simulink model "myLIN_F16Block"  (Simulink 7.6)
settings: Solver=ode5  StartTime=0.0  StopTime=100  FixedStep=0.001  RelTol=1e-3
values from neighbouring files (symbols this model uses):
  dLEF = 0    [F16Data.mat]    (also in F16LinmodTestData.m; F16NolinearModelInitialData.m; F16NolinearModelRemoveWindControlData_low.m; F16hi_7500_394_all.mat)
  fi_flag_Simulink = 0    [F16Data.mat]    (also in F16hi_7500_394_all.mat; F16lo_7500_394_all.mat; myFindF16Dynamics.m; runLINF16sim.m)
  trim_control_hi = [-2.97973164861 0.00874607850104 0.0680302158183]    [F16Data.mat]    (also in F16hi_7500_394_all.mat = [-1.41046812571 -0.0839337172095 -0.0125601395798]; F16lo_7500_394_all.mat = [-1.41046812571 -0.0839337172095 -0.0125601395798])
  trim_control_lo = [-1.5494258131 -1.24450697103e-10 -4.77959844983e-09]    [F16Data.mat]    (also in F16hi_7500_394_all.mat = [-1.08947517229 0.155794241881 0.128606760221]; F16lo_7500_394_all.mat = [-1.64183174326 -4.38546100082e-10 -1.68300124238e-08])
  trim_state_lin = [0 0 9843 0 1.13910469244e-17 0 393.72 1.13910469244e-17 0 0 0 0]    [F16Data.mat]    (also in F16hi_7500_394_all.mat = [0 0 7500 0 0.000279617532986 0 394 0.000279617532986 0 0 0 ; F16lo_7500_394_all.mat = [0 0 7500 0 0.0237311750075 0 394 0.0237311750075 0 0 0 0]; myFindF16Dynamics.m = trim_state_lo; runLINF16sim.m = trim_state_lo)
  trim_thrust_hi = 2279.08519955    [F16Data.mat]    (also in F16hi_7500_394_all.mat = -26942.451508; F16lo_7500_394_all.mat = -26942.451508)
  trim_thrust_lo = -206727.459732    [F16Data.mat]    (also in F16hi_7500_394_all.mat = 1004.07804585; F16lo_7500_394_all.mat = -98159.5668651)
settings Model: Creator=keviczky  LastModifiedBy=WhisPer  ExtModeAutoUpdateStatusClock=off
settings DataIOCC: Decimation=50  LimitDataPoints=off  SignalLoggingName=sigsOut
settings OptimizationCC: BooleanDataType=off
settings DebuggingCC: SaveWithParameterizedLinksMsg=none  SignalResolutionControl=TryResolveAllWithWarning  SolverPrmCheckMsg=none  MultiTaskDSMMsg=warning  MultiTaskCondExecSysMsg=none  StrictBusMsg=None
settings HardwareCC: TargetUnknown=on
settings RTWCC: IncludeERTFirstTime=on

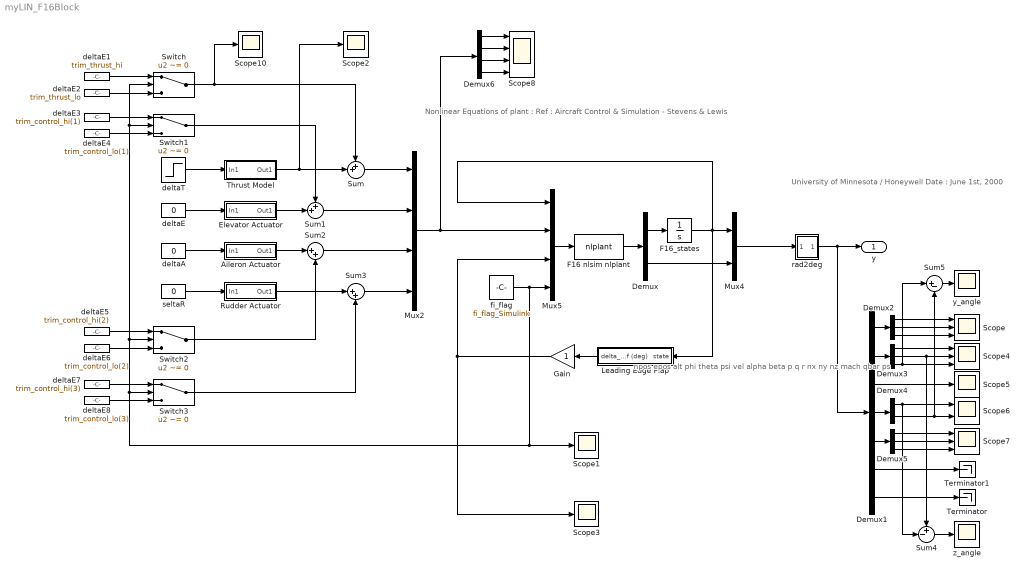
== system myLIN_F16Block ==
  note: npos
      | epos
      | alt
      | phi
      | theta
      | psi
      | vel
      | alpha
      | beta
      | p
      | q
      | r
      | nx
      | ny
      | nz
      | mach
      | qbar
      | ps
  note: University of Minnesota / Honeywell
      | Date : June 1st, 2000
  note: Nonlinear Equations of plant :
      | Ref : Aircraft Control & Simulation
      | - Stevens & Lewis
  Aileron Actuator : Subsystem  AncestorBlock=F16_Actuator_Library/Aileron Actuator
  Demux : Demux  Outputs=[12 6]
  Demux1 : Demux  Outputs=[3 3 1 2 3 3 3]
  Demux2 : Demux  Outputs=3
  Demux3 : Demux  Outputs=3
  Demux4 : Demux  Outputs=2
  Demux5 : Demux  Outputs=3
  Demux6 : Demux
  Elevator Actuator : Subsystem  AncestorBlock=F16_Actuator_Library/Elevator Actuator
  F16 nlsim nlplant : MATLABFcn  MATLABFcn=nlplant  OutputDimensions=18  OutputSignalType=real
  F16_states : Integrator  InitialCondition=trim_state_lin
  Gain : Gain
  Leading Edge Flap : Subsystem
  Mux2 : Mux
  Mux4 : Mux  Inputs=2
  Mux5 : Mux  Inputs=[12 4 1 1]
  Rudder Actuator : Subsystem  AncestorBlock=F16_Actuator_Library/Rudder Actuator
  Scope : Scope  NumInputPorts=3
      settings: YMin=-9000~-4e-008~2000  YMax=3000~1.6e-007~9500
  Scope{1..3,5,10} (5 alike) : Scope
      Scope1 settings: YMin=0  YMax=3500
      Scope10 settings: YMin=0  YMax=3500  SaveName=ScopeData12
      Scope2 settings: YMin=0  YMax=3500  SaveName=ScopeData2
      Scope3 settings: YMin=-13.5  YMax=-9  SaveName=ScopeData3
      Scope5 settings: YMin=-13.5  YMax=-9  SaveName=ScopeData5
  Scope4 : Scope  NumInputPorts=3
      settings: YMin=-9000~-4e-008~2000  YMax=3000~1.6e-007~9500  SaveName=ScopeData4
  Scope6 : Scope  NumInputPorts=2
      settings: YMin=-9000~-4e-008  YMax=3000~1.6e-007  SaveName=ScopeData6
  Scope7 : Scope  NumInputPorts=3
      settings: YMin=-9000~-4e-008~2000  YMax=3000~1.6e-007~9500  SaveName=ScopeData7
  Scope8 : Scope  NumInputPorts=4
      settings: YMin=-9000~-4e-008~2000~-5  YMax=3000~1.6e-007~9500~5  SaveName=ScopeData8
  Sum : Sum  Inputs=++|
  Sum1 : Sum  Inputs=++|
  Sum2 : Sum  Inputs=|++
  Sum3 : Sum  Inputs=|++
  Sum4 : Sum  Inputs=+-|
  Sum5 : Sum  Inputs=|+-
  Switch{,1..3} (4 alike) : Switch  Criteria=u2 ~= 0
  Terminator : Terminator
  Terminator1 : Terminator
  Thrust Model : Subsystem  AncestorBlock=F16_Actuator_Library/Thrust Model
  deltaA : Constant  Value=0
  deltaE : Constant  Value=0
  deltaE1 : Constant  Value=trim_thrust_hi
  deltaE2 : Constant  Value=trim_thrust_lo
  deltaE3 : Constant  Value=trim_control_hi(1)
  deltaE4 : Constant  Value=trim_control_lo(1)
  deltaE5 : Constant  Value=trim_control_hi(2)
  deltaE6 : Constant  Value=trim_control_lo(2)
  deltaE7 : Constant  Value=trim_control_hi(3)
  deltaE8 : Constant  Value=trim_control_lo(3)
  deltaT : Step  Time=5  After=0  SampleTime=0
  fi_flag : Constant  Value=fi_flag_Simulink
  rad2deg : Subsystem
  seltaR : Constant  Value=0
  y_angle : Scope
      settings: YMin=0  YMax=3500  SaveName=ScopeData10
  z_angle : Scope
      settings: YMin=0  YMax=3500  SaveName=ScopeData9
  y : Outport
  wires:
  Mux4/1 -> rad2deg/1(In1)
  F16 nlsim nlplant/1 -> Demux/1
  Demux/1 -> F16_states/1
  Demux/2 -> Mux4/2
  Mux5/1 -> F16 nlsim nlplant/1
  Mux2/1 -> Mux5/2, Demux6/1
  rad2deg/1(Out1) -> y/1, Demux1/1
  F16_states/1 -> Mux4/1, Mux5/1, Leading Edge Flap/1(state)
  fi_flag/1 -> Mux5/4, Scope1/1, Switch3/2, Switch2/2, Switch/2, Switch1/2
  Leading Edge Flap/1(delta_lef (deg)) -> Gain/1
  Demux1/1 -> Demux2/1
  Demux2/1 -> Scope/1
  Demux2/2 -> Scope/2
  Demux2/3 -> Scope/3
  Demux1/7 -> Terminator/1
  deltaE1/1 -> Switch/1
  deltaE2/1 -> Switch/3
  deltaE3/1 -> Switch1/1
  deltaE4/1 -> Switch1/3
  deltaE5/1 -> Switch2/1
  deltaE6/1 -> Switch2/3
  deltaE7/1 -> Switch3/1
  deltaE8/1 -> Switch3/3
  seltaR/1 -> Rudder Actuator/1(In1)
  deltaA/1 -> Aileron Actuator/1(In1)
  deltaE/1 -> Elevator Actuator/1(In1)
  deltaT/1 -> Thrust Model/1(In1)
  Elevator Actuator/1(Out1) -> Sum1/2
  Sum1/1 -> Mux2/2
  Sum/1 -> Mux2/1
  Thrust Model/1(Out1) -> Sum/2, Scope2/1
  Sum3/1 -> Mux2/4
  Rudder Actuator/1(Out1) -> Sum3/1
  Aileron Actuator/1(Out1) -> Sum2/1
  Sum2/1 -> Mux2/3
  Demux3/1 -> Scope4/1
  Demux3/2 -> Scope4/2, Sum4/1
  Demux3/3 -> Scope4/3, Sum5/1
  Demux1/2 -> Demux3/1
  Demux1/3 -> Scope5/1
  Demux1/4 -> Demux4/1
  Demux4/1 -> Scope6/1, Sum4/2
  Demux4/2 -> Scope6/2, Sum5/2
  Demux5/1 -> Scope7/1
  Demux5/2 -> Scope7/2
  Demux5/3 -> Scope7/3
  Demux1/5 -> Demux5/1
  Demux1/6 -> Terminator1/1
  Demux6/1 -> Scope8/1
  Demux6/2 -> Scope8/2
  Demux6/3 -> Scope8/3
  Demux6/4 -> Scope8/4
  Switch/1 -> Sum/1, Scope10/1
  Switch1/1 -> Sum1/1
  Sum4/1 -> z_angle/1
  Sum5/1 -> y_angle/1
  Gain/1 -> Mux5/3, Scope3/1
  Switch2/1 -> Sum2/2
  Switch3/1 -> Sum3/2

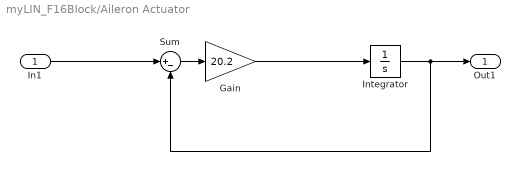
== system myLIN_F16Block/Aileron Actuator ==
  In1 : Inport
  Gain : Gain  Gain=20.2  SaturateOnIntegerOverflow=on  OutDataTypeStr=Inherit: Same as input  ParamDataTypeStr=Inherit: Same as input
  "Integrator " : Integrator  UpperSaturationLimit=21.5  LowerSaturationLimit=-21.5
  Sum : Sum  Inputs=|+-  SaturateOnIntegerOverflow=on  InputSameDT=on  OutDataTypeStr=Inherit: Same as first input
  Out1 : Outport
  wires:
  "Integrator "/1 -> Sum/2, Out1/1
  Gain/1 -> "Integrator "/1
  Sum/1 -> Gain/1
  In1/1 -> Sum/1

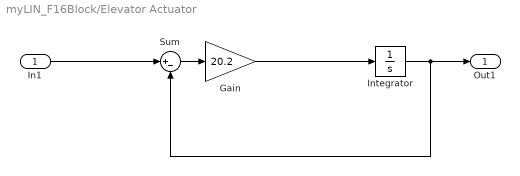
== system myLIN_F16Block/Elevator Actuator ==
  In1 : Inport
  Gain : Gain  Gain=20.2  SaturateOnIntegerOverflow=on  OutDataTypeStr=Inherit: Same as input  ParamDataTypeStr=Inherit: Same as input
  "Integrator " : Integrator  UpperSaturationLimit=25  LowerSaturationLimit=-25
  Sum : Sum  Inputs=|+-  SaturateOnIntegerOverflow=on  InputSameDT=on  OutDataTypeStr=Inherit: Same as first input
  Out1 : Outport
  wires:
  "Integrator "/1 -> Sum/2, Out1/1
  Gain/1 -> "Integrator "/1
  Sum/1 -> Gain/1
  In1/1 -> Sum/1

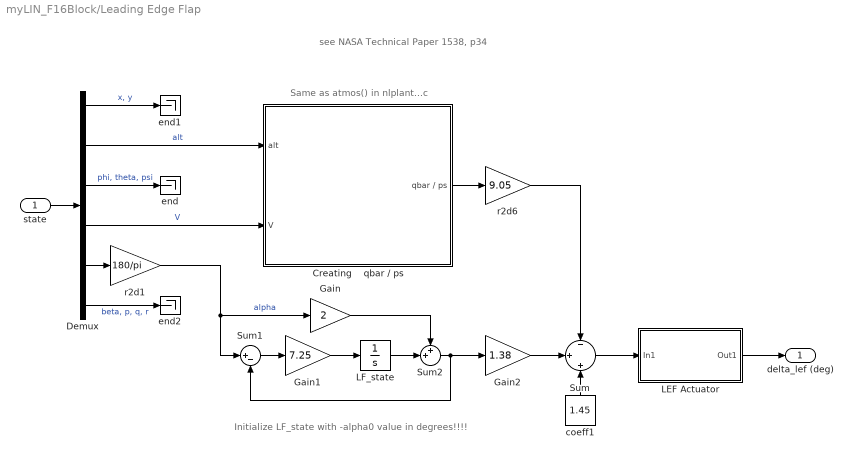
== system myLIN_F16Block/Leading Edge Flap ==
  note: see NASA Technical Paper 1538, p34
  note: Same as atmos() in nlplant...c
  note: Initialize LF_state with -alpha0 value in degrees!!!!
  state : Inport
  Creating    qbar / ps : Subsystem
  Demux : Demux  Outputs=[2,1,3,1,1,4]
  Gain : Gain  Gain=2  SaturateOnIntegerOverflow=on  OutDataTypeStr=Inherit: Same as input  ParamDataTypeStr=Inherit: Same as input
  Gain1 : Gain  Gain=7.25  SaturateOnIntegerOverflow=on  OutDataTypeStr=Inherit: Same as input  ParamDataTypeStr=Inherit: Same as input
  Gain2 : Gain  Gain=1.38  SaturateOnIntegerOverflow=on  OutDataTypeStr=Inherit: Same as input  ParamDataTypeStr=Inherit: Same as input
  LEF Actuator : Subsystem  AncestorBlock=F16_Actuator_Library/Aileron Actuator
  LF_state : Integrator  InitialCondition=-trim_state_lin(8)*180/pi
  Sum : Sum  Inputs=-|+|+  SaturateOnIntegerOverflow=on  InputSameDT=on  OutDataTypeStr=Inherit: Same as first input
  Sum1 : Sum  Inputs=|+-  SaturateOnIntegerOverflow=on  InputSameDT=on  OutDataTypeStr=Inherit: Same as first input
  Sum2 : Sum  Inputs=++|  SaturateOnIntegerOverflow=on  InputSameDT=on  OutDataTypeStr=Inherit: Same as first input
  coeff1 : Constant  Value=1.45
  end : Terminator
  end1 : Terminator
  end2 : Terminator
  r2d1 : Gain  Gain=180/pi  SaturateOnIntegerOverflow=on  OutDataTypeStr=Inherit: Same as input  ParamDataTypeStr=Inherit: Same as input
  r2d6 : Gain  Gain=9.05  SaturateOnIntegerOverflow=on  OutDataTypeStr=Inherit: Same as input  ParamDataTypeStr=Inherit: Same as input
  delta_lef (deg) : Outport
  wires:
  LEF Actuator/1(Out1) -> delta_lef (deg)/1
  Sum/1 -> LEF Actuator/1(In1)
  Demux/3 -> end/1  "phi, theta, psi"
  state/1 -> Demux/1
  Sum1/1 -> Gain1/1
  Gain1/1 -> LF_state/1
  Gain/1 -> Sum2/1
  Gain2/1 -> Sum/2
  Demux/1 -> end1/1  "x, y"
  Demux/5 -> r2d1/1
  Demux/6 -> end2/1  "beta, p, q, r"
  coeff1/1 -> Sum/3
  Sum2/1 -> Sum1/2, Gain2/1
  LF_state/1 -> Sum2/2
  r2d1/1 -> Sum1/1, Gain/1  "alpha"
  Demux/4 -> Creating    qbar / ps/2(V)  "V"
  Creating    qbar / ps/1(qbar / ps) -> r2d6/1
  r2d6/1 -> Sum/1
  Demux/2 -> Creating    qbar / ps/1(alt)  "alt"

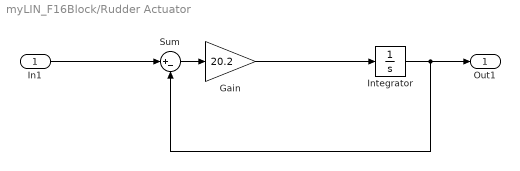
== system myLIN_F16Block/Rudder Actuator ==
  In1 : Inport
  Gain : Gain  Gain=20.2  SaturateOnIntegerOverflow=on  OutDataTypeStr=Inherit: Same as input  ParamDataTypeStr=Inherit: Same as input
  "Integrator " : Integrator  UpperSaturationLimit=30  LowerSaturationLimit=-30
  Sum : Sum  Inputs=|+-  SaturateOnIntegerOverflow=on  InputSameDT=on  OutDataTypeStr=Inherit: Same as first input
  Out1 : Outport
  wires:
  "Integrator "/1 -> Sum/2, Out1/1
  Gain/1 -> "Integrator "/1
  Sum/1 -> Gain/1
  In1/1 -> Sum/1

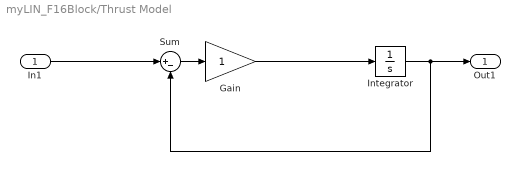
== system myLIN_F16Block/Thrust Model ==
  In1 : Inport
  Gain : Gain  SaturateOnIntegerOverflow=on  OutDataTypeStr=Inherit: Same as input  ParamDataTypeStr=Inherit: Same as input
  "Integrator " : Integrator  UpperSaturationLimit=30  LowerSaturationLimit=-30
  Sum : Sum  Inputs=|+-  SaturateOnIntegerOverflow=on  InputSameDT=on  OutDataTypeStr=Inherit: Same as first input
  Out1 : Outport
  wires:
  "Integrator "/1 -> Sum/2, Out1/1
  Gain/1 -> "Integrator "/1
  Sum/1 -> Gain/1
  In1/1 -> Sum/1

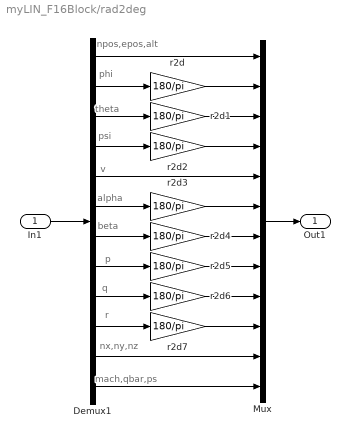
== system myLIN_F16Block/rad2deg ==
  note: npos,epos,alt
  note: phi
  note: theta
  note: psi
  note: v
  note: alpha
  note: beta
  note: p
  note: q
  note: r
  note: nx,ny,nz
  note: mach,qbar,ps
  In1 : Inport
  Demux1 : Demux  Outputs=[3 1 1 1 1 1 1 1 1 1 3 3]
  Mux : Mux  Inputs=[3 1 1 1 1 1 1 1 1 1 3 3]
  r2d{,1..7} (8 alike) : Gain  Gain=180/pi  SaturateOnIntegerOverflow=on  OutDataTypeStr=Inherit: Same as input  ParamDataTypeStr=Inherit: Same as input
  Out1 : Outport
  wires:
  In1/1 -> Demux1/1
  Demux1/2 -> r2d/1
  Demux1/3 -> r2d1/1
  Demux1/4 -> r2d2/1
  Demux1/1 -> Mux/1
  Demux1/5 -> Mux/5
  r2d2/1 -> Mux/4
  r2d1/1 -> Mux/3
  r2d/1 -> Mux/2
  Demux1/6 -> r2d3/1
  Demux1/7 -> r2d4/1
  Demux1/8 -> r2d5/1
  Demux1/9 -> r2d6/1
  Demux1/10 -> r2d7/1
  r2d3/1 -> Mux/6
  r2d4/1 -> Mux/7
  r2d5/1 -> Mux/8
  r2d6/1 -> Mux/9
  r2d7/1 -> Mux/10
  Mux/1 -> Out1/1
  Demux1/11 -> Mux/11
  Demux1/12 -> Mux/12

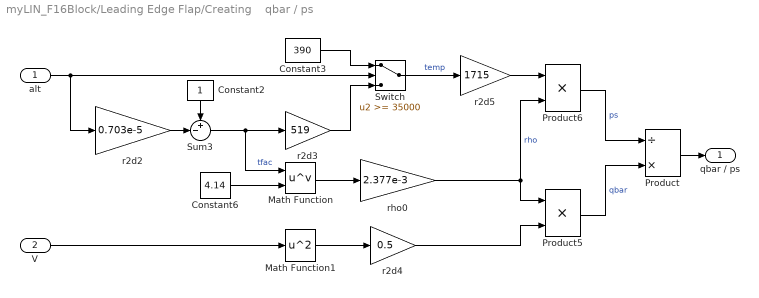
== system myLIN_F16Block/Leading Edge Flap/Creating    qbar / ps ==
  alt : Inport
  V : Inport  Port=2
  Constant2 : Constant
  Constant3 : Constant  Value=390
  Constant6 : Constant  Value=4.14
  Math Function : Math  Operator=pow  SaturateOnIntegerOverflow=on
  Math Function1 : Math  Operator=square  SaturateOnIntegerOverflow=on
  Product : Product  Inputs=/*  SaturateOnIntegerOverflow=on  InputSameDT=on  OutDataTypeStr=Inherit: Same as first input
  Product5 : Product  Inputs=**  SaturateOnIntegerOverflow=on  InputSameDT=on  OutDataTypeStr=Inherit: Same as first input
  Product6 : Product  Inputs=**  SaturateOnIntegerOverflow=on  InputSameDT=on  OutDataTypeStr=Inherit: Same as first input
  Sum3 : Sum  Inputs=+-|  SaturateOnIntegerOverflow=on  InputSameDT=on  OutDataTypeStr=Inherit: Same as first input
  Switch : Switch  Threshold=35000  SaturateOnIntegerOverflow=on  InputSameDT=on
  r2d2 : Gain  Gain=0.703e-5  SaturateOnIntegerOverflow=on  OutDataTypeStr=Inherit: Same as input  ParamDataTypeStr=Inherit: Same as input
  r2d3 : Gain  Gain=519  SaturateOnIntegerOverflow=on  OutDataTypeStr=Inherit: Same as input  ParamDataTypeStr=Inherit: Same as input
  r2d4 : Gain  Gain=0.5  SaturateOnIntegerOverflow=on  OutDataTypeStr=Inherit: Same as input  ParamDataTypeStr=Inherit: Same as input
  r2d5 : Gain  Gain=1715  SaturateOnIntegerOverflow=on  OutDataTypeStr=Inherit: Same as input  ParamDataTypeStr=Inherit: Same as input
  rho0 : Gain  Gain=2.377e-3  SaturateOnIntegerOverflow=on  OutDataTypeStr=Inherit: Same as input  ParamDataTypeStr=Inherit: Same as input
  qbar / ps : Outport
  wires:
  alt/1 -> r2d2/1, Switch/2
  Sum3/1 -> Math Function/1, r2d3/1  "tfac"
  Constant3/1 -> Switch/1
  r2d3/1 -> Switch/3
  Constant6/1 -> Math Function/2
  rho0/1 -> Product5/1, Product6/2  "rho"
  Math Function1/1 -> r2d4/1
  r2d2/1 -> Sum3/2
  Constant2/1 -> Sum3/1
  Math Function/1 -> rho0/1
  r2d4/1 -> Product5/2
  Switch/1 -> r2d5/1  "temp"
  r2d5/1 -> Product6/1
  Product6/1 -> Product/1  "ps"
  Product5/1 -> Product/2  "qbar"
  Product/1 -> qbar / ps/1
  V/1 -> Math Function1/1

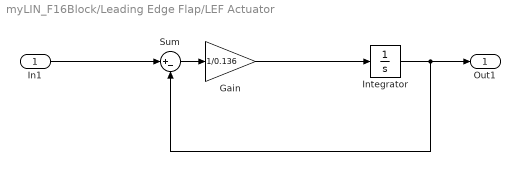
== system myLIN_F16Block/Leading Edge Flap/LEF Actuator ==
  In1 : Inport
  Gain : Gain  Gain=1/0.136  SaturateOnIntegerOverflow=on  OutDataTypeStr=Inherit: Same as input  ParamDataTypeStr=Inherit: Same as input
  "Integrator " : Integrator  InitialCondition=dLEF  UpperSaturationLimit=21.5  LowerSaturationLimit=-21.5
  Sum : Sum  Inputs=|+-  SaturateOnIntegerOverflow=on  InputSameDT=on  OutDataTypeStr=Inherit: Same as first input
  Out1 : Outport
  wires:
  "Integrator "/1 -> Sum/2, Out1/1
  Gain/1 -> "Integrator "/1
  Sum/1 -> Gain/1
  In1/1 -> Sum/1
